simulink model "F16version1"  (R2023b)
settings: Solver=VariableStepAuto  StartTime=0.0  StopTime=60  FixedStep=0.1  RelTol=1e-3
libraries: simulink_extras x4, simulink x2, aerolibasang x2, shared6dof x1, aerolibanim x1
(part 1 of 2)
settings Model: Creator=TADTAWAN  LastModifiedBy=TADTAWAN

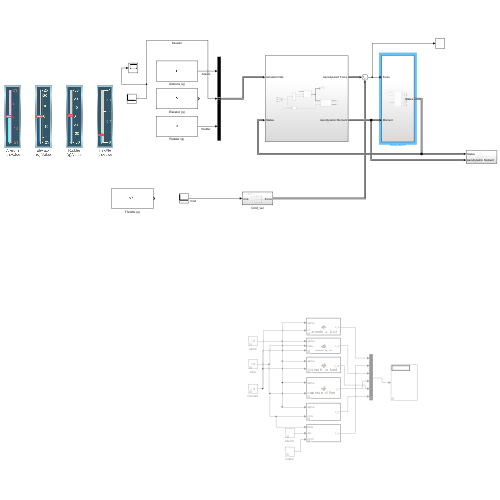
[thumbnail: Simulink's stored preview of the top-level diagram]
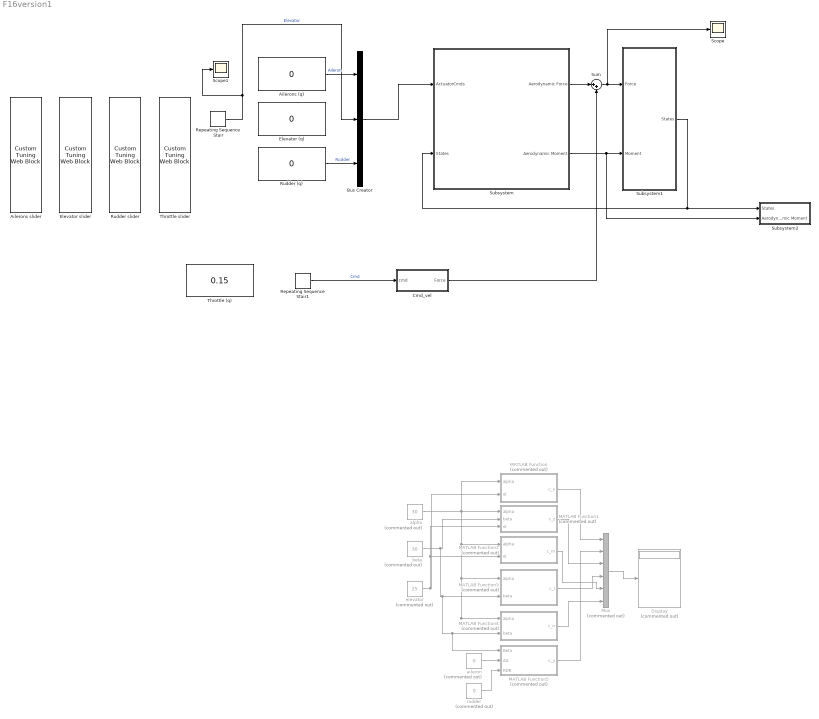
== system F16version1 ==
  Ailerons (q) : Constant  Value=0
  Ailerons slider : CustomTuningWebBlock  LabelPosition=Bottom  ShowInitialText=on  Configuration="{\"components\":[{\"name\":\"LinearScaleComponent\",\"settings\":{\"bounds\":{\"max\":21.5,\"min\":-21.5,\"tickInterval\":\"auto\"},\"internalTickHeightScaleFactor\":0.5,\"labelColor\":[181,82,43],\"labelFont\":{\"font\":\"Arial\",\"fontSize\":12},\"labelOffset\":0.05,\"labelTransparency\":1,\"needleImage\":{\"size\":[596,842],\"src\":\"data:image\\/svg+xml;base64,PD94bWwgdmVyc2lvbj0iMS4wIiBlbmNvZGluZz0idXRmLTgiPz4NCjwhLS0gR2VuZXJhdG9yOiBBZG9iZSBJbGx1c3RyYXRvciAyNS4wLjAsIFNWRyBFeHBvcnQgUGx1Zy1JbiAuIFNWRyBWZXJzaW9uOiA2LjAwIEJ1aWxkIDApICAtLT4NCjxzdmcgdmVyc2lvbj0iMS4xIg0KCSBpZD0ic3ZnOCIgeG1sbnM6Y2M9Imh0dHA6Ly9jcmVhdGl2ZWNvbW1vbnMub3JnL25zIyIgeG1sbnM6ZGM9Imh0dHA6Ly9wdXJsLm9yZy9kYy9lbGVtZW50cy8xLjEvIiB4bWxuczppbmtzY2FwZT0iaHR0cDovL3d3dy5pbmtzY2FwZS5vcmcvbmFtZXNw ...(+2420 chars)\",\"srcOrientation\":\"horizontal\"},\"needleOffset\":[0.0642123287671233,-0.8044596912521441],\"needleSize\":{\"height\":0.07668067226890757,\"width\":0.4337797619047619},\"position\":[0.03623949579831933,0.2829861111111111,0.6088789682539683,0.9196428571428571],\"referencePoint\":\"auto\",\"scaleColors\":[],\"scaleColorsSize\":0.2,\"scaleDirection\":\"BT\",\"showLabels\":1,\"showMinorTicks\":0,\"showSpanLine\":1,\"showTicks\":1,\"tickColor\":[150,61,168],\"tickTransparency\":1,\"valueBarColor\":[15,255,255],\"valueBarOffset\":-0.27,\"valueBarSize\":0.1,\"valueBarTransparency\":1}},{\"name\":\"BackgroundImageComponent\",\"settings\":{\"image\":{\"size\":[380,101],\"src\":\"data:image\\/svg+xml;base64,PHN2ZyB4bWxucz0iaHR0cDovL3d3dy53My5vcmcvMjAwMC9zdmciIHhtbG5zOnhsaW5rPSJodHRwOi8vd3d3LnczLm9yZy8xOTk5L3hsaW5rIiB2aWV3Qm94PSIwIDAgMzgwIDEwMSI+PGRlZnM+PHN0eWxlPi5jbHMtMXtmaWxsOiMwMDJiNDI7fS5jbHMtMntmaWxsOiM0MjcwODI7fS5jbHMtM3tmaWxsOnVybCgjcmFkaWFsLWdyYWRpZW50KTt9LmNscy00e2ZpbGw6I2M4YzhjODtzdHJva2U6IzAwMDt9PC9zdHlsZT48cmFkaWFsR3JhZGllbnQgaWQ9InJhZGlhbC1ncmFkaWVudCIgY3g9IjE5MCIgY3k9IjUwLjUiIHI9IjI2OS4yMSIgZ3JhZGllbnRVbml0cz0idXNlclNwYWNlT25Vc2UiPjxzdG9wIG9mZnNldD0iMC4wMSIgc3RvcC1jb2xvcj0iIzNlNGY1OCIvPjxzdG9wIG9mZnNldD0iMC4wNiIgc3RvcC1jb2xvcj0iIzQ0NTc2MSIvPjxzdG9wIG9mZnNldD0iMC4xNSIgc3RvcC1jb2xvcj0iIzU1NmE3NiIvPjxzdG9wIG9mZnNldD0iMC4yNSIgc3RvcC1jb2xvcj0iIzZkODg5NSIvPjxzdG9wIG9mZnNldD0iMC4zOCIgc3RvcC1jb2xvcj0iIzhmYjJjMyIvPjxzdG9wIG9mZnNldD0iMC41MiIgc3RvcC1jb2xvcj0iI2I2ZTRmYSIvPjxzdG9wIG9mZnNldD0iMSIgc3RvcC1jb2xvcj0iIzE1NDY1NyIvPjwvcmFkaWFsR3JhZGllbnQ+PC9kZWZzPjxnIGlkPSJmcmFtZSI+PGcgaWQ9IkxheWVyXzIiIGRhdGEtbmFtZT0iTGF5ZXIgMiI+PGcgaWQ9IkxheWVyXzEtMiIgZGF0YS1uYW1lPSJMYXllciAxLTIiPjxyZWN0IGlkPSJyZWN0MTAzNiIgY2xhc3M9ImNscy0xIiB4PSIxMSIgeT0iMTEiIHdpZHRoPSIzNTgiIGhlaWdodD0iNzkiLz48cGF0aCBpZD0icGF0aDEwMzgiIGNsYXNzPSJjbHMtMiIgZD0iTTgsOFY5M0gzNzJWOFpNMzY5LDkwSDExVjExSDM2OVoiLz48cGF0aCBpZD0icGF0aDEwNDAiIGNsYXNzPSJjbHMtMyIgZD0iTTAsMFYxMDFIMzgwVjBaTTM3Miw5M0g4VjhIMzcyWiIvPjwvZz48L2c+PC9nPjxnIGlkPSJ0cmFjayI+PHBhdGggaWQ9InJlY3QxNjExIiBjbGFzcz0iY2xzLTQiIGQ9Ik0zMy4zNywyNi41OUgzNDYuNjNjNCwwLDcuMjUsMi42LDcuMjUsNS44MWgwYzAsMy4yMS0zLjI1LDUuODItNy4yNSw1LjgySDMzLjM3Yy00LDAtNy4yNS0yLjYxLTcuMjUtNS44MmgwQzI2LjEyLDI5LjE5LDI5LjM3LDI2LjU5LDMzLjM3LDI2LjU5WiIvPjwvZz48L3N2Zz4=\",\"srcOrientation\":\"horizontal\"},\"position\":[0,0,1,1],\"scaleMode\":\"0\"}},{\"name\":\"ForegroundImageComponent\",\"settings\":{\"image\":{\"size\":[0,0],\"src\":\"default\",\"srcOrientation\":[]},\"isForeground\":1,\"position\":[0,0,1,1],\"scaleMode\":\"0\"}}],\"settings\":{\"BindingType\":\"param\",\"aspectRatio\":3.7777777777777777,\"backgroundColor\":[0,0,0,\"1\"],\"backgroundOffset\":0,\"backgroundOpacity\":1,\"fixedAspectRatio\":\"on\",\"foregroundColor\":[252,252,196],\"orientation\":\"vertical\",\"showBackgroundColor\":false,\"value\":0,\"version\":\"R2023a\"},\"type\":\"LinearGauge\"}"
  Bus Creator : BusCreator  Inputs=3
  Cmd_vel : Subsystem
  Display : Display  Commented=on
  Elevator (q) : Constant  Value=0
  Elevator slider : CustomTuningWebBlock  LabelPosition=Bottom  ShowInitialText=on  Configuration="{\"components\":[{\"name\":\"LinearScaleComponent\",\"settings\":{\"bounds\":{\"max\":25,\"min\":-25,\"tickInterval\":\"auto\"},\"internalTickHeightScaleFactor\":0.5,\"labelColor\":[255,255,200],\"labelFont\":{\"font\":\"Arial\",\"fontSize\":12},\"labelOffset\":0.05,\"labelTransparency\":1,\"needleImage\":{\"size\":[596,842],\"src\":\"data:image\\/svg+xml;base64,PD94bWwgdmVyc2lvbj0iMS4wIiBlbmNvZGluZz0idXRmLTgiPz4NCjwhLS0gR2VuZXJhdG9yOiBBZG9iZSBJbGx1c3RyYXRvciAyNS4wLjAsIFNWRyBFeHBvcnQgUGx1Zy1JbiAuIFNWRyBWZXJzaW9uOiA2LjAwIEJ1aWxkIDApICAtLT4NCjxzdmcgdmVyc2lvbj0iMS4xIg0KCSBpZD0ic3ZnOCIgeG1sbnM6Y2M9Imh0dHA6Ly9jcmVhdGl2ZWNvbW1vbnMub3JnL25zIyIgeG1sbnM6ZGM9Imh0dHA6Ly9wdXJsLm9yZy9kYy9lbGVtZW50cy8xLjEvIiB4bWxuczppbmtzY2FwZT0iaHR0cDovL3d3dy5pbmtzY2FwZS5vcmcvbmFtZXNw ...(+2420 chars)\",\"srcOrientation\":\"horizontal\"},\"needleOffset\":[0.0642123287671233,-0.8044596912521441],\"needleSize\":{\"height\":0.07668067226890757,\"width\":0.4337797619047619},\"position\":[0.03623949579831933,0.2829861111111111,0.6088789682539683,0.9196428571428571],\"referencePoint\":\"auto\",\"scaleColors\":[],\"scaleColorsSize\":0.2,\"scaleDirection\":\"BT\",\"showLabels\":1,\"showMinorTicks\":0,\"showSpanLine\":1,\"showTicks\":1,\"tickColor\":[252,252,197],\"tickTransparency\":1,\"valueBarColor\":[0,114,189],\"valueBarOffset\":-0.27,\"valueBarSize\":0.1,\"valueBarTransparency\":1}},{\"name\":\"BackgroundImageComponent\",\"settings\":{\"image\":{\"size\":[380,101],\"src\":\"data:image\\/svg+xml;base64,PHN2ZyB4bWxucz0iaHR0cDovL3d3dy53My5vcmcvMjAwMC9zdmciIHhtbG5zOnhsaW5rPSJodHRwOi8vd3d3LnczLm9yZy8xOTk5L3hsaW5rIiB2aWV3Qm94PSIwIDAgMzgwIDEwMSI+PGRlZnM+PHN0eWxlPi5jbHMtMXtmaWxsOiMwMDJiNDI7fS5jbHMtMntmaWxsOiM0MjcwODI7fS5jbHMtM3tmaWxsOnVybCgjcmFkaWFsLWdyYWRpZW50KTt9LmNscy00e2ZpbGw6I2M4YzhjODtzdHJva2U6IzAwMDt9PC9zdHlsZT48cmFkaWFsR3JhZGllbnQgaWQ9InJhZGlhbC1ncmFkaWVudCIgY3g9IjE5MCIgY3k9IjUwLjUiIHI9IjI2OS4yMSIgZ3JhZGllbnRVbml0cz0idXNlclNwYWNlT25Vc2UiPjxzdG9wIG9mZnNldD0iMC4wMSIgc3RvcC1jb2xvcj0iIzNlNGY1OCIvPjxzdG9wIG9mZnNldD0iMC4wNiIgc3RvcC1jb2xvcj0iIzQ0NTc2MSIvPjxzdG9wIG9mZnNldD0iMC4xNSIgc3RvcC1jb2xvcj0iIzU1NmE3NiIvPjxzdG9wIG9mZnNldD0iMC4yNSIgc3RvcC1jb2xvcj0iIzZkODg5NSIvPjxzdG9wIG9mZnNldD0iMC4zOCIgc3RvcC1jb2xvcj0iIzhmYjJjMyIvPjxzdG9wIG9mZnNldD0iMC41MiIgc3RvcC1jb2xvcj0iI2I2ZTRmYSIvPjxzdG9wIG9mZnNldD0iMSIgc3RvcC1jb2xvcj0iIzE1NDY1NyIvPjwvcmFkaWFsR3JhZGllbnQ+PC9kZWZzPjxnIGlkPSJmcmFtZSI+PGcgaWQ9IkxheWVyXzIiIGRhdGEtbmFtZT0iTGF5ZXIgMiI+PGcgaWQ9IkxheWVyXzEtMiIgZGF0YS1uYW1lPSJMYXllciAxLTIiPjxyZWN0IGlkPSJyZWN0MTAzNiIgY2xhc3M9ImNscy0xIiB4PSIxMSIgeT0iMTEiIHdpZHRoPSIzNTgiIGhlaWdodD0iNzkiLz48cGF0aCBpZD0icGF0aDEwMzgiIGNsYXNzPSJjbHMtMiIgZD0iTTgsOFY5M0gzNzJWOFpNMzY5LDkwSDExVjExSDM2OVoiLz48cGF0aCBpZD0icGF0aDEwNDAiIGNsYXNzPSJjbHMtMyIgZD0iTTAsMFYxMDFIMzgwVjBaTTM3Miw5M0g4VjhIMzcyWiIvPjwvZz48L2c+PC9nPjxnIGlkPSJ0cmFjayI+PHBhdGggaWQ9InJlY3QxNjExIiBjbGFzcz0iY2xzLTQiIGQ9Ik0zMy4zNywyNi41OUgzNDYuNjNjNCwwLDcuMjUsMi42LDcuMjUsNS44MWgwYzAsMy4yMS0zLjI1LDUuODItNy4yNSw1LjgySDMzLjM3Yy00LDAtNy4yNS0yLjYxLTcuMjUtNS44MmgwQzI2LjEyLDI5LjE5LDI5LjM3LDI2LjU5LDMzLjM3LDI2LjU5WiIvPjwvZz48L3N2Zz4=\",\"srcOrientation\":\"horizontal\"},\"position\":[0,0,1,1],\"scaleMode\":\"0\"}},{\"name\":\"ForegroundImageComponent\",\"settings\":{\"image\":{\"size\":[0,0],\"src\":\"default\",\"srcOrientation\":[]},\"isForeground\":1,\"position\":[0,0,1,1],\"scaleMode\":\"0\"}}],\"settings\":{\"BindingType\":\"param\",\"aspectRatio\":3.7777777777777777,\"backgroundColor\":[0,0,0,\"1\"],\"backgroundOffset\":0,\"backgroundOpacity\":1,\"fixedAspectRatio\":\"on\",\"foregroundColor\":[252,252,196],\"orientation\":\"vertical\",\"showBackgroundColor\":false,\"value\":0,\"version\":\"R2023a\"},\"type\":\"LinearGauge\"}"
  MATLAB Function : MATLAB Function  Commented=on  TreatAsAtomicUnit=on
  MATLAB Function1 : MATLAB Function  Commented=on  TreatAsAtomicUnit=on
  MATLAB Function2 : MATLAB Function  Commented=on  TreatAsAtomicUnit=on
  MATLAB Function3 : MATLAB Function  Commented=on  TreatAsAtomicUnit=on
  MATLAB Function4 : MATLAB Function  Commented=on  TreatAsAtomicUnit=on
  MATLAB Function5 : MATLAB Function  Commented=on  TreatAsAtomicUnit=on
  Mux : Mux  Commented=on  Inputs=6
  Repeating Sequence Stair : simulink/Sources/Repeating Sequence Stair  OutValues=[-1.5].'  tsamp=10  OutMin=[]  OutMax=[]  OutDataTypeStr=double  OutputDataTypeScalingMode=double  OutDataType=fixdt(0,8)  ConRadixGroup=Best Precision: Vector-wise  OutScaling=2^-12
  Repeating Sequence Stair1 : simulink/Sources/Repeating Sequence Stair  OutValues=[0.5].'  tsamp=10  OutMin=[]  OutMax=[]  OutDataTypeStr=double  OutputDataTypeScalingMode=double  OutDataType=fixdt(0,8)  ConRadixGroup=Best Precision: Vector-wise  OutScaling=2^-12
  Rudder (q) : Constant  Value=0
  Rudder slider : CustomTuningWebBlock  LabelPosition=Bottom  ShowInitialText=on  Configuration="{\"components\":[{\"name\":\"LinearScaleComponent\",\"settings\":{\"bounds\":{\"max\":30,\"min\":-30,\"tickInterval\":\"auto\"},\"internalTickHeightScaleFactor\":0.5,\"labelColor\":[255,255,200],\"labelFont\":{\"font\":\"Arial\",\"fontSize\":12},\"labelOffset\":0.05,\"labelTransparency\":1,\"needleImage\":{\"size\":[596,842],\"src\":\"data:image\\/svg+xml;base64,PD94bWwgdmVyc2lvbj0iMS4wIiBlbmNvZGluZz0idXRmLTgiPz4NCjwhLS0gR2VuZXJhdG9yOiBBZG9iZSBJbGx1c3RyYXRvciAyNS4wLjAsIFNWRyBFeHBvcnQgUGx1Zy1JbiAuIFNWRyBWZXJzaW9uOiA2LjAwIEJ1aWxkIDApICAtLT4NCjxzdmcgdmVyc2lvbj0iMS4xIg0KCSBpZD0ic3ZnOCIgeG1sbnM6Y2M9Imh0dHA6Ly9jcmVhdGl2ZWNvbW1vbnMub3JnL25zIyIgeG1sbnM6ZGM9Imh0dHA6Ly9wdXJsLm9yZy9kYy9lbGVtZW50cy8xLjEvIiB4bWxuczppbmtzY2FwZT0iaHR0cDovL3d3dy5pbmtzY2FwZS5vcmcvbmFtZXNw ...(+2420 chars)\",\"srcOrientation\":\"Right\"},\"needleOffset\":[-0.21513706793802145,-0.7877922077922078],\"needleSize\":{\"height\":0.07666301169590643,\"width\":0.43370508054522927},\"position\":[0.03623949579831933,0.2829861111111111,0.6088789682539683,0.9196428571428571],\"referencePoint\":\"auto\",\"scaleColors\":[],\"scaleColorsSize\":0.2,\"scaleDirection\":\"BT\",\"showLabels\":1,\"showMinorTicks\":0,\"showSpanLine\":1,\"showTicks\":1,\"tickColor\":[252,252,197],\"tickTransparency\":1,\"valueBarColor\":[0,114,189],\"valueBarOffset\":-0.27,\"valueBarSize\":0.1,\"valueBarTransparency\":1}},{\"name\":\"BackgroundImageComponent\",\"settings\":{\"image\":{\"size\":[380,101],\"src\":\"data:image\\/svg+xml;base64,PHN2ZyB4bWxucz0iaHR0cDovL3d3dy53My5vcmcvMjAwMC9zdmciIHhtbG5zOnhsaW5rPSJodHRwOi8vd3d3LnczLm9yZy8xOTk5L3hsaW5rIiB2aWV3Qm94PSIwIDAgMzgwIDEwMSI+PGRlZnM+PHN0eWxlPi5jbHMtMXtmaWxsOiMwMDJiNDI7fS5jbHMtMntmaWxsOiM0MjcwODI7fS5jbHMtM3tmaWxsOnVybCgjcmFkaWFsLWdyYWRpZW50KTt9LmNscy00e2ZpbGw6I2M4YzhjODtzdHJva2U6IzAwMDt9PC9zdHlsZT48cmFkaWFsR3JhZGllbnQgaWQ9InJhZGlhbC1ncmFkaWVudCIgY3g9IjE5MCIgY3k9IjUwLjUiIHI9IjI2OS4yMSIgZ3JhZGllbnRVbml0cz0idXNlclNwYWNlT25Vc2UiPjxzdG9wIG9mZnNldD0iMC4wMSIgc3RvcC1jb2xvcj0iIzNlNGY1OCIvPjxzdG9wIG9mZnNldD0iMC4wNiIgc3RvcC1jb2xvcj0iIzQ0NTc2MSIvPjxzdG9wIG9mZnNldD0iMC4xNSIgc3RvcC1jb2xvcj0iIzU1NmE3NiIvPjxzdG9wIG9mZnNldD0iMC4yNSIgc3RvcC1jb2xvcj0iIzZkODg5NSIvPjxzdG9wIG9mZnNldD0iMC4zOCIgc3RvcC1jb2xvcj0iIzhmYjJjMyIvPjxzdG9wIG9mZnNldD0iMC41MiIgc3RvcC1jb2xvcj0iI2I2ZTRmYSIvPjxzdG9wIG9mZnNldD0iMSIgc3RvcC1jb2xvcj0iIzE1NDY1NyIvPjwvcmFkaWFsR3JhZGllbnQ+PC9kZWZzPjxnIGlkPSJmcmFtZSI+PGcgaWQ9IkxheWVyXzIiIGRhdGEtbmFtZT0iTGF5ZXIgMiI+PGcgaWQ9IkxheWVyXzEtMiIgZGF0YS1uYW1lPSJMYXllciAxLTIiPjxyZWN0IGlkPSJyZWN0MTAzNiIgY2xhc3M9ImNscy0xIiB4PSIxMSIgeT0iMTEiIHdpZHRoPSIzNTgiIGhlaWdodD0iNzkiLz48cGF0aCBpZD0icGF0aDEwMzgiIGNsYXNzPSJjbHMtMiIgZD0iTTgsOFY5M0gzNzJWOFpNMzY5LDkwSDExVjExSDM2OVoiLz48cGF0aCBpZD0icGF0aDEwNDAiIGNsYXNzPSJjbHMtMyIgZD0iTTAsMFYxMDFIMzgwVjBaTTM3Miw5M0g4VjhIMzcyWiIvPjwvZz48L2c+PC9nPjxnIGlkPSJ0cmFjayI+PHBhdGggaWQ9InJlY3QxNjExIiBjbGFzcz0iY2xzLTQiIGQ9Ik0zMy4zNywyNi41OUgzNDYuNjNjNCwwLDcuMjUsMi42LDcuMjUsNS44MWgwYzAsMy4yMS0zLjI1LDUuODItNy4yNSw1LjgySDMzLjM3Yy00LDAtNy4yNS0yLjYxLTcuMjUtNS44MmgwQzI2LjEyLDI5LjE5LDI5LjM3LDI2LjU5LDMzLjM3LDI2LjU5WiIvPjwvZz48L3N2Zz4=\",\"srcOrientation\":\"horizontal\"},\"position\":[0,0,1,1],\"scaleMode\":\"0\"}},{\"name\":\"ForegroundImageComponent\",\"settings\":{\"image\":{\"size\":[0,0],\"src\":\"default\",\"srcOrientation\":[]},\"isForeground\":1,\"position\":[0,0,1,1],\"scaleMode\":\"0\"}}],\"settings\":{\"BindingType\":\"param\",\"aspectRatio\":3.7777777777777777,\"backgroundColor\":[0,0,0,\"1\"],\"backgroundOffset\":0,\"backgroundOpacity\":1,\"fixedAspectRatio\":\"on\",\"foregroundColor\":[252,252,196],\"orientation\":\"vertical\",\"showBackgroundColor\":false,\"value\":0,\"version\":\"R2023a\"},\"type\":\"LinearGauge\"}"
  Scope : Scope
  Scope1 : Scope
  Subsystem : Subsystem
  Subsystem1 : Subsystem
  Subsystem2 : Subsystem
  Sum : Sum  Inputs=|++
  Throttle (q) : Constant  Value=0.15
  Throttle slider : CustomTuningWebBlock  LabelPosition=Bottom  ShowInitialText=on  Configuration="{\"components\":[{\"name\":\"LinearScaleComponent\",\"settings\":{\"bounds\":{\"max\":1,\"min\":0,\"tickInterval\":\"auto\"},\"internalTickHeightScaleFactor\":0.5,\"labelColor\":[255,255,200],\"labelFont\":{\"font\":\"Arial\",\"fontSize\":12},\"labelOffset\":0.05,\"labelTransparency\":1,\"needleImage\":{\"size\":[596,842],\"src\":\"data:image\\/svg+xml;base64,PD94bWwgdmVyc2lvbj0iMS4wIiBlbmNvZGluZz0idXRmLTgiPz4NCjwhLS0gR2VuZXJhdG9yOiBBZG9iZSBJbGx1c3RyYXRvciAyNS4wLjAsIFNWRyBFeHBvcnQgUGx1Zy1JbiAuIFNWRyBWZXJzaW9uOiA2LjAwIEJ1aWxkIDApICAtLT4NCjxzdmcgdmVyc2lvbj0iMS4xIg0KCSBpZD0ic3ZnOCIgeG1sbnM6Y2M9Imh0dHA6Ly9jcmVhdGl2ZWNvbW1vbnMub3JnL25zIyIgeG1sbnM6ZGM9Imh0dHA6Ly9wdXJsLm9yZy9kYy9lbGVtZW50cy8xLjEvIiB4bWxuczppbmtzY2FwZT0iaHR0cDovL3d3dy5pbmtzY2FwZS5vcmcvbmFtZXNw ...(+2420 chars)\",\"srcOrientation\":\"horizontal\"},\"needleOffset\":[0.0642123287671233,-0.8044596912521441],\"needleSize\":{\"height\":0.07668067226890757,\"width\":0.4337797619047619},\"position\":[0.03623949579831933,0.2829861111111111,0.6088789682539683,0.9196428571428571],\"referencePoint\":\"auto\",\"scaleColors\":[],\"scaleColorsSize\":0.2,\"scaleDirection\":\"BT\",\"showLabels\":1,\"showMinorTicks\":0,\"showSpanLine\":1,\"showTicks\":1,\"tickColor\":[252,252,197],\"tickTransparency\":1,\"valueBarColor\":[0,114,189],\"valueBarOffset\":-0.27,\"valueBarSize\":0.1,\"valueBarTransparency\":1}},{\"name\":\"BackgroundImageComponent\",\"settings\":{\"image\":{\"size\":[380,101],\"src\":\"data:image\\/svg+xml;base64,PHN2ZyB4bWxucz0iaHR0cDovL3d3dy53My5vcmcvMjAwMC9zdmciIHhtbG5zOnhsaW5rPSJodHRwOi8vd3d3LnczLm9yZy8xOTk5L3hsaW5rIiB2aWV3Qm94PSIwIDAgMzgwIDEwMSI+PGRlZnM+PHN0eWxlPi5jbHMtMXtmaWxsOiMwMDJiNDI7fS5jbHMtMntmaWxsOiM0MjcwODI7fS5jbHMtM3tmaWxsOnVybCgjcmFkaWFsLWdyYWRpZW50KTt9LmNscy00e2ZpbGw6I2M4YzhjODtzdHJva2U6IzAwMDt9PC9zdHlsZT48cmFkaWFsR3JhZGllbnQgaWQ9InJhZGlhbC1ncmFkaWVudCIgY3g9IjE5MCIgY3k9IjUwLjUiIHI9IjI2OS4yMSIgZ3JhZGllbnRVbml0cz0idXNlclNwYWNlT25Vc2UiPjxzdG9wIG9mZnNldD0iMC4wMSIgc3RvcC1jb2xvcj0iIzNlNGY1OCIvPjxzdG9wIG9mZnNldD0iMC4wNiIgc3RvcC1jb2xvcj0iIzQ0NTc2MSIvPjxzdG9wIG9mZnNldD0iMC4xNSIgc3RvcC1jb2xvcj0iIzU1NmE3NiIvPjxzdG9wIG9mZnNldD0iMC4yNSIgc3RvcC1jb2xvcj0iIzZkODg5NSIvPjxzdG9wIG9mZnNldD0iMC4zOCIgc3RvcC1jb2xvcj0iIzhmYjJjMyIvPjxzdG9wIG9mZnNldD0iMC41MiIgc3RvcC1jb2xvcj0iI2I2ZTRmYSIvPjxzdG9wIG9mZnNldD0iMSIgc3RvcC1jb2xvcj0iIzE1NDY1NyIvPjwvcmFkaWFsR3JhZGllbnQ+PC9kZWZzPjxnIGlkPSJmcmFtZSI+PGcgaWQ9IkxheWVyXzIiIGRhdGEtbmFtZT0iTGF5ZXIgMiI+PGcgaWQ9IkxheWVyXzEtMiIgZGF0YS1uYW1lPSJMYXllciAxLTIiPjxyZWN0IGlkPSJyZWN0MTAzNiIgY2xhc3M9ImNscy0xIiB4PSIxMSIgeT0iMTEiIHdpZHRoPSIzNTgiIGhlaWdodD0iNzkiLz48cGF0aCBpZD0icGF0aDEwMzgiIGNsYXNzPSJjbHMtMiIgZD0iTTgsOFY5M0gzNzJWOFpNMzY5LDkwSDExVjExSDM2OVoiLz48cGF0aCBpZD0icGF0aDEwNDAiIGNsYXNzPSJjbHMtMyIgZD0iTTAsMFYxMDFIMzgwVjBaTTM3Miw5M0g4VjhIMzcyWiIvPjwvZz48L2c+PC9nPjxnIGlkPSJ0cmFjayI+PHBhdGggaWQ9InJlY3QxNjExIiBjbGFzcz0iY2xzLTQiIGQ9Ik0zMy4zNywyNi41OUgzNDYuNjNjNCwwLDcuMjUsMi42LDcuMjUsNS44MWgwYzAsMy4yMS0zLjI1LDUuODItNy4yNSw1LjgySDMzLjM3Yy00LDAtNy4yNS0yLjYxLTcuMjUtNS44MmgwQzI2LjEyLDI5LjE5LDI5LjM3LDI2LjU5LDMzLjM3LDI2LjU5WiIvPjwvZz48L3N2Zz4=\",\"srcOrientation\":\"horizontal\"},\"position\":[0,0,1,1],\"scaleMode\":\"0\"}},{\"name\":\"ForegroundImageComponent\",\"settings\":{\"image\":{\"size\":[0,0],\"src\":\"default\",\"srcOrientation\":[]},\"isForeground\":1,\"position\":[0,0,1,1],\"scaleMode\":\"0\"}}],\"settings\":{\"BindingType\":\"param\",\"aspectRatio\":3.7777777777777777,\"backgroundColor\":[0,0,0,\"1\"],\"backgroundOffset\":0,\"backgroundOpacity\":1,\"fixedAspectRatio\":\"on\",\"foregroundColor\":[252,252,196],\"orientation\":\"vertical\",\"showBackgroundColor\":false,\"value\":0,\"version\":\"R2023a\"},\"type\":\"LinearGauge\"}"
  aileron : Constant  Commented=on  Value=0
  alpha : Constant  Commented=on  Value=30
  beta : Constant  Commented=on  Value=30
  elevator : Constant  Commented=on  Value=25
  rudder : Constant  Commented=on  Value=0
  wires:
  Ailerons (q)/1 -> Bus Creator/1  "Aileron"
  Rudder (q)/1 -> Bus Creator/3  "Rudder"
  Bus Creator/1 -> Subsystem/1(ActuatorCmds)
  Subsystem/1(Aerodynamic Force) -> Sum/1
  Subsystem/2(Aerodynamic Moment) -> Subsystem2/2(Aerodynamic Moment), Subsystem1/2(Moment)
  Cmd_vel/1(Force) -> Sum/2
  Sum/1 -> Scope/1, Subsystem1/1(Force)
  Subsystem1/1(States) -> Subsystem/2(States), Subsystem2/1(States)
  alpha/1 -> MATLAB Function4/1(alpha), MATLAB Function3/1(alpha), MATLAB Function2/1(alpha), MATLAB Function1/1(alpha), MATLAB Function/1(alpha)
  beta/1 -> MATLAB Function5/1(Beta), MATLAB Function4/2(beta), MATLAB Function3/2(beta), MATLAB Function1/2(beta)
  elevator/1 -> MATLAB Function2/2(el), MATLAB Function1/3(el), MATLAB Function/2(el)
  aileron/1 -> MATLAB Function5/2(AIL)
  rudder/1 -> MATLAB Function5/3(RDR)
  MATLAB Function/1(c_x) -> Mux/1
  MATLAB Function5/1(c_y) -> Mux/2
  MATLAB Function1/1(c_z) -> Mux/3
  MATLAB Function3/1(c_l) -> Mux/4
  MATLAB Function2/1(c_m) -> Mux/5
  MATLAB Function4/1(c_n) -> Mux/6
  Mux/1 -> Display/1
  Repeating Sequence Stair/1 -> Scope1/1, Bus Creator/2  "Elevator"
  Repeating Sequence Stair1/1 -> Cmd_vel/1(cmd)  "Cmd"

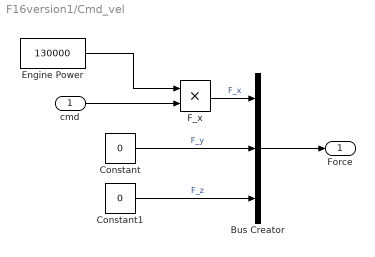
== system F16version1/Cmd_vel ==
  cmd : Inport
  Bus Creator : BusCreator  Inputs=3
  Constant : Constant  Value=0
  Constant1 : Constant  Value=0
  Engine Power : Constant  Value=130000
  F_x : Product
  Force : Outport
  wires:
  Engine Power/1 -> F_x/1
  cmd/1 -> F_x/2
  F_x/1 -> Bus Creator/1  "F_x"
  Constant/1 -> Bus Creator/2  "F_y"
  Constant1/1 -> Bus Creator/3  "F_z"
  Bus Creator/1 -> Force/1

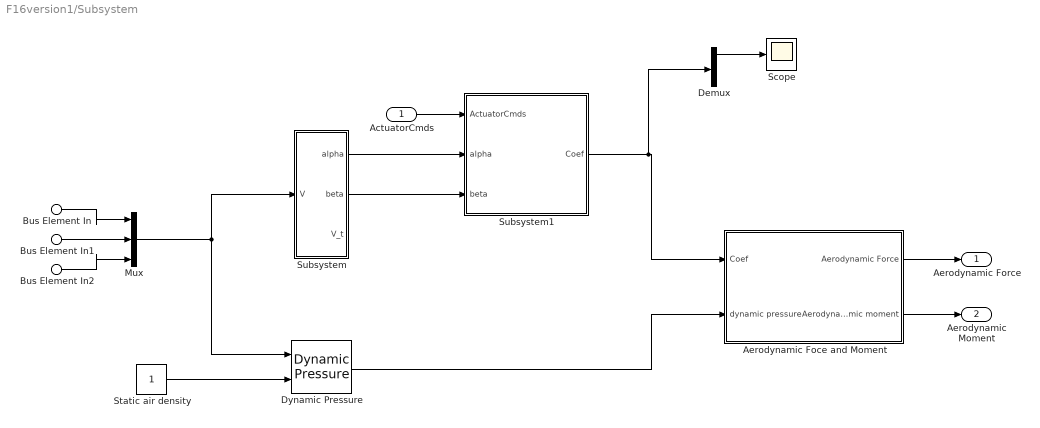
== system F16version1/Subsystem ==
  ActuatorCmds : Inport
  Bus Element In : Inport  Port=2  PortName=States  Element=U
  Bus Element In1 : Inport  Port=2  PortName=States  Element=V
  Bus Element In2 : Inport  Port=2  PortName=States  Element=W
  Aerodynamic Foce and Moment : Subsystem
  Demux : Demux  Outputs=6
  Dynamic Pressure : aerolibasang/Dynamic Pressure
  Mux : Mux  Inputs=3
  Scope : Scope
  Static air density : Constant
  Subsystem : Subsystem
  Subsystem1 : Subsystem
  Aerodynamic Force : Outport
  Aerodynamic Moment : Outport  Port=2
  wires:
  Bus Element In1/1 -> Mux/2
  Bus Element In/1 -> Mux/1
  Bus Element In2/1 -> Mux/3
  Mux/1 -> Dynamic Pressure/1, Subsystem/1(V)
  ActuatorCmds/1 -> Subsystem1/1(ActuatorCmds)
  Subsystem/1(alpha) -> Subsystem1/2(alpha)
  Subsystem/2(beta) -> Subsystem1/3(beta)
  Static air density/1 -> Dynamic Pressure/2
  Dynamic Pressure/1 -> Aerodynamic Foce and Moment/2(dynamic pressure)
  Subsystem1/1(Coef) -> Demux/1, Aerodynamic Foce and Moment/1(Coef)
  Aerodynamic Foce and Moment/1(Aerodynamic Force) -> Aerodynamic Force/1
  Aerodynamic Foce and Moment/2(Aerodynamic moment) -> Aerodynamic Moment/1
  Demux/1 -> Scope/1

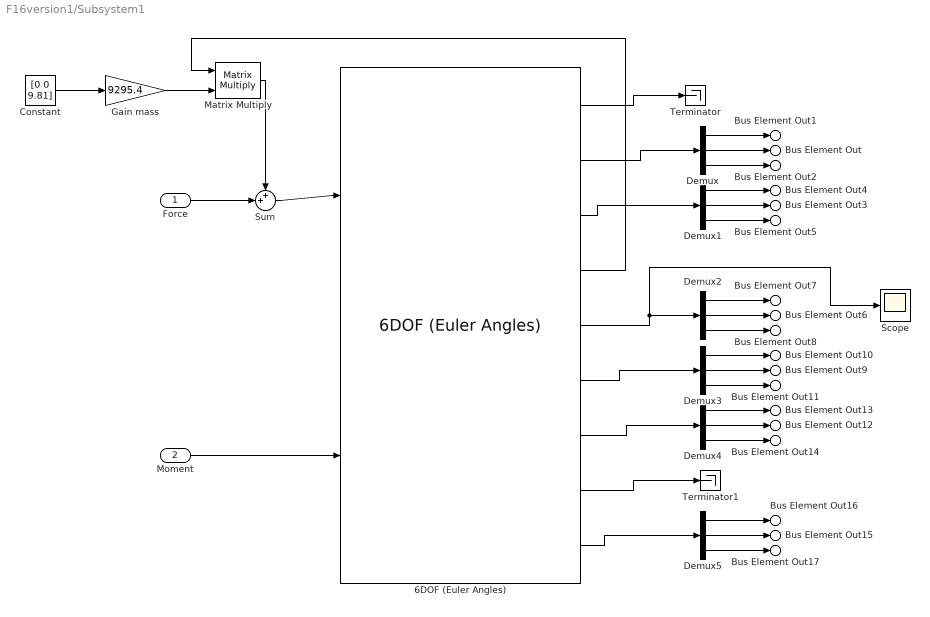
== system F16version1/Subsystem1 ==
  Force : Inport
  Moment : Inport  Port=2
  6DOF (Euler Angles) : shared6dof/6DOF (Euler Angles)  units=Metric (MKS)  mtype=Fixed  rep=Euler Angles  xme_0=[0, 0,-2000]  Vm_0=[0.01, 0.01, 0.01]  eul_0=[0.0, 0.0, 0]  pm_0=[0, 0, 0]  mass_0=91188/9.81  mass_e=0.5  mass_f=2.0  inertia=|  inertia_e=eye(3)  inertia_f=2*eye(3)  k_quat=1.0  vre_flag=off  abi_flag=on  aMode=0  xme_statename={'Xe', 'Ye', 'Ze'}  Vm_statename={'U', 'V', 'W'}  eul_statename={'phi', 'theta', 'psi'}  quat_statename=''  pm_statename={'p', 'q', 'r'}  mass_statename=''
      | [12881.4, 0, 1522.0;
      |  0, 75696.9, 0;
      |  1522.0, 0, 85557.2]
  Constant : Constant  Value=[0 0 9.81]
  Demux{,1..5} (6 alike) : Demux  Outputs=3
  Gain mass : Gain  Gain=9295.4
  Matrix Multiply : Product  Multiplication=Matrix(*)
  Scope : Scope
  Sum : Sum  Inputs=++|
  Terminator : Terminator
  Terminator1 : Terminator
  Bus Element Out : Outport  PortName=States  Element=Ye
  Bus Element Out1 : Outport  PortName=States  Element=Xe
  Bus Element Out2 : Outport  PortName=States  Element=Ze
  Bus Element Out3 : Outport  PortName=States  Element=theta
  Bus Element Out4 : Outport  PortName=States  Element=phi
  Bus Element Out5 : Outport  PortName=States  Element=psi
  Bus Element Out6 : Outport  PortName=States  Element=V
  Bus Element Out7 : Outport  PortName=States  Element=U
  Bus Element Out8 : Outport  PortName=States  Element=W
  Bus Element Out9 : Outport  PortName=States  Element=q
  Bus Element Out10 : Outport  PortName=States  Element=p
  Bus Element Out11 : Outport  PortName=States  Element=r
  Bus Element Out12 : Outport  PortName=States  Element=q_dot
  Bus Element Out13 : Outport  PortName=States  Element=p_dot
  Bus Element Out14 : Outport  PortName=States  Element=r_dot
  Bus Element Out15 : Outport  PortName=States  Element=Aye
  Bus Element Out16 : Outport  PortName=States  Element=Axe
  Bus Element Out17 : Outport  PortName=States  Element=Aze
  wires:
  Moment/1 -> 6DOF (Euler Angles)/2
  Force/1 -> Sum/2
  Constant/1 -> Gain mass/1
  Gain mass/1 -> Matrix Multiply/2
  Matrix Multiply/1 -> Sum/1
  Sum/1 -> 6DOF (Euler Angles)/1
  6DOF (Euler Angles)/4 -> Matrix Multiply/1
  6DOF (Euler Angles)/2 -> Demux/1
  Demux/2 -> Bus Element Out/1
  Demux/1 -> Bus Element Out1/1
  Demux/3 -> Bus Element Out2/1
  Demux1/3 -> Bus Element Out5/1
  Demux1/2 -> Bus Element Out3/1
  Demux1/1 -> Bus Element Out4/1
  6DOF (Euler Angles)/3 -> Demux1/1
  Demux2/1 -> Bus Element Out7/1
  Demux2/3 -> Bus Element Out8/1
  Demux2/2 -> Bus Element Out6/1
  6DOF (Euler Angles)/5 -> Scope/1, Demux2/1
  Demux3/1 -> Bus Element Out10/1
  Demux3/3 -> Bus Element Out11/1
  Demux3/2 -> Bus Element Out9/1
  6DOF (Euler Angles)/6 -> Demux3/1
  Demux4/1 -> Bus Element Out13/1
  Demux4/3 -> Bus Element Out14/1
  Demux4/2 -> Bus Element Out12/1
  6DOF (Euler Angles)/7 -> Demux4/1
  Demux5/1 -> Bus Element Out16/1
  Demux5/3 -> Bus Element Out17/1
  Demux5/2 -> Bus Element Out15/1
  6DOF (Euler Angles)/1 -> Terminator/1
  6DOF (Euler Angles)/8 -> Terminator1/1
  6DOF (Euler Angles)/9 -> Demux5/1

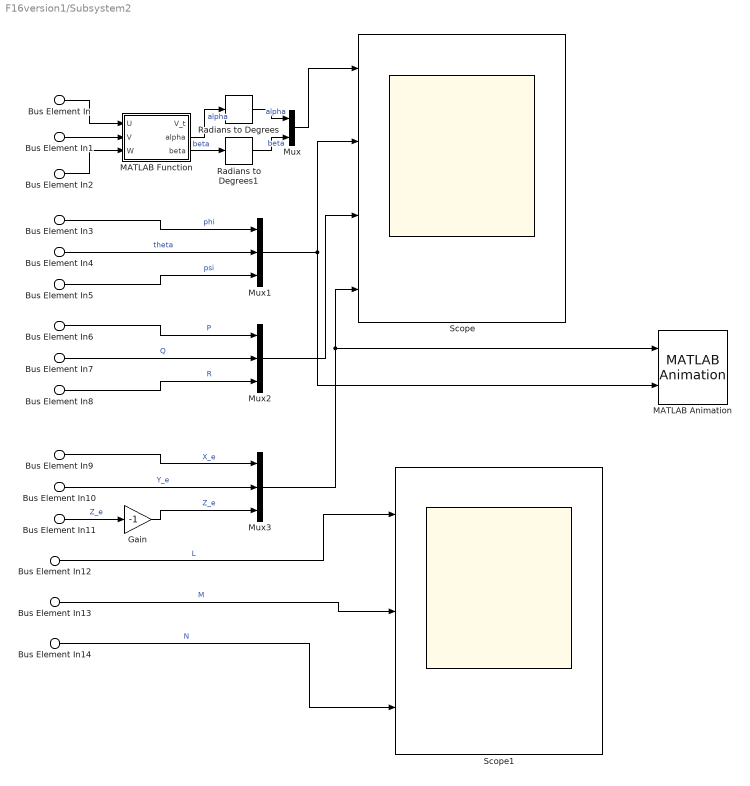
== system F16version1/Subsystem2 ==
  Bus Element In : Inport  PortName=States  Element=U
  Bus Element In2 : Inport  PortName=States  Element=W
  Bus Element In1 : Inport  PortName=States  Element=V
  Bus Element In3 : Inport  PortName=States  Element=phi
  Bus Element In4 : Inport  PortName=States  Element=theta
  Bus Element In5 : Inport  PortName=States  Element=psi
  Bus Element In6 : Inport  PortName=States  Element=p
  Bus Element In7 : Inport  PortName=States  Element=q
  Bus Element In8 : Inport  PortName=States  Element=r
  Bus Element In9 : Inport  PortName=States  Element=Xe
  Bus Element In10 : Inport  PortName=States  Element=Ye
  Bus Element In11 : Inport  PortName=States  Element=Ze
  Bus Element In12 : Inport  Port=2  PortName=Aerodynamic Moment  Element=L
  Bus Element In13 : Inport  Port=2  PortName=Aerodynamic Moment  Element=M
  Bus Element In14 : Inport  Port=2  PortName=Aerodynamic Moment  Element=N
  Gain : Gain  Gain=-1
  MATLAB Animation : aerolibanim/MATLAB Animation  Tag=Matlab Animation 6 DOF  Vehicles=1  Geometries='astredwedge.mat'  BoundingBoxCoordinates=[-50,50,-50,50,-50,50]  CameraOffset=[-150,-50,0]  CameraViewAngle=3  SampleTime=0.2  FigurePosition=[-1020,327,559,396]
  MATLAB Function : MATLAB Function  TreatAsAtomicUnit=on
  Mux : Mux  Inputs=2
  Mux1 : Mux  Inputs=3
  Mux2 : Mux  Inputs=3
  Mux3 : Mux  Inputs=3
  Radians to Degrees : simulink_extras/Transformations/Radians to Degrees
  Radians to Degrees1 : simulink_extras/Transformations/Radians to Degrees
  Scope : Scope  NumInputPorts=4
  Scope1 : Scope  NumInputPorts=3
  wires:
  Bus Element In/1 -> MATLAB Function/1(U)
  Bus Element In1/1 -> MATLAB Function/2(V)
  Bus Element In2/1 -> MATLAB Function/3(W)
  MATLAB Function/2(alpha) -> Radians to Degrees/1  "alpha"
  MATLAB Function/3(beta) -> Radians to Degrees1/1  "beta"
  Mux/1 -> Scope/1
  Bus Element In4/1 -> Mux1/2  "theta"
  Bus Element In3/1 -> Mux1/1  "phi"
  Bus Element In5/1 -> Mux1/3  "psi"
  Mux1/1 -> MATLAB Animation/2, Scope/2
  Bus Element In8/1 -> Mux2/3  "R"
  Bus Element In7/1 -> Mux2/2  "Q"
  Mux2/1 -> Scope/3
  Bus Element In6/1 -> Mux2/1  "P"
  Bus Element In11/1 -> Gain/1  "Z_e"
  Bus Element In10/1 -> Mux3/2  "Y_e"
  Bus Element In9/1 -> Mux3/1  "X_e"
  Mux3/1 -> MATLAB Animation/1, Scope/4
  Bus Element In13/1 -> Scope1/2  "M"
  Bus Element In12/1 -> Scope1/1  "L"
  Bus Element In14/1 -> Scope1/3  "N"
  Radians to Degrees/1 -> Mux/1  "alpha"
  Radians to Degrees1/1 -> Mux/2  "beta"
  Gain/1 -> Mux3/3  "Z_e"

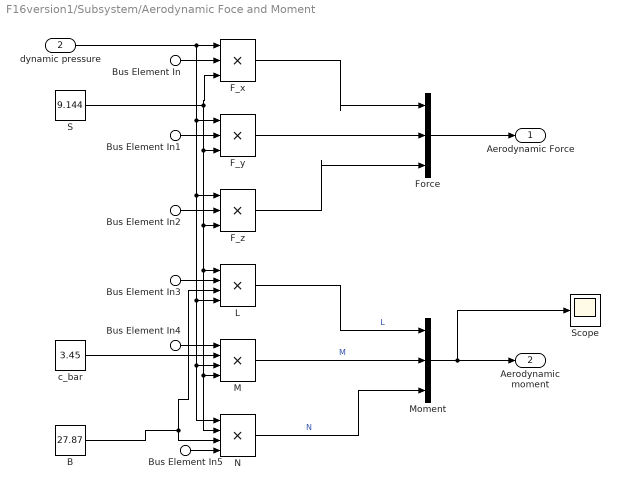
== system F16version1/Subsystem/Aerodynamic Foce and Moment ==
  Bus Element In : Inport  PortName=Coef  Element=c_x
  Bus Element In1 : Inport  PortName=Coef  Element=c_y
  Bus Element In2 : Inport  PortName=Coef  Element=c_z
  Bus Element In3 : Inport  PortName=Coef  Element=c_l
  Bus Element In4 : Inport  PortName=Coef  Element=c_m
  Bus Element In5 : Inport  PortName=Coef  Element=c_n
  dynamic pressure : Inport  Port=2
  B : Constant  Value=27.87
  F_x : Product  Inputs=3
  F_y : Product  Inputs=3
  F_z : Product  Inputs=3
  Force : BusCreator  Inputs=3
  L : Product  Inputs=4
  M : Product  Inputs=4
  Moment : BusCreator  Inputs=3
  N : Product  Inputs=4
  S : Constant  Value=9.144
  Scope : Scope
  c_bar : Constant  Value=3.45
  Aerodynamic Force : Outport
  Aerodynamic moment : Outport  Port=2
  wires:
  dynamic pressure/1 -> F_y/1, L/4, N/1, M/3, F_z/1, F_x/1
  Bus Element In/1 -> F_x/2
  S/1 -> F_x/3, L/1, N/2, M/4, F_z/3, F_y/3
  Bus Element In1/1 -> F_y/2
  Bus Element In2/1 -> F_z/2
  c_bar/1 -> M/2
  Bus Element In3/1 -> L/2
  Bus Element In4/1 -> M/1
  Bus Element In5/1 -> N/4
  B/1 -> N/3, L/3
  F_x/1 -> Force/1
  F_y/1 -> Force/2
  F_z/1 -> Force/3
  L/1 -> Moment/1  "L"
  M/1 -> Moment/2  "M"
  N/1 -> Moment/3  "N"
  Force/1 -> Aerodynamic Force/1
  Moment/1 -> Scope/1, Aerodynamic moment/1

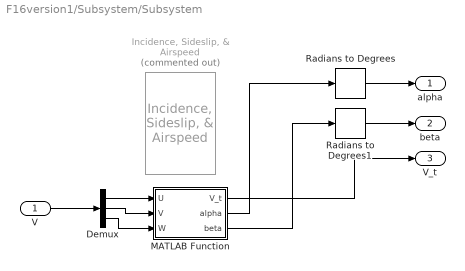
== system F16version1/Subsystem/Subsystem ==
  V : Inport
  Demux : Demux  Outputs=3
  "Incidence, Sideslip, & Airspeed" : aerolibasang/Incidence, Sideslip, & Airspeed  Commented=on
  MATLAB Function : MATLAB Function  TreatAsAtomicUnit=on
  Radians to Degrees : simulink_extras/Transformations/Radians to Degrees
  Radians to Degrees1 : simulink_extras/Transformations/Radians to Degrees
  alpha : Outport
  beta : Outport  Port=2
  V_t : Outport  Port=3
  wires:
  V/1 -> Demux/1
  Demux/1 -> MATLAB Function/1(U)
  Demux/2 -> MATLAB Function/2(V)
  Demux/3 -> MATLAB Function/3(W)
  Radians to Degrees/1 -> alpha/1
  Radians to Degrees1/1 -> beta/1
  MATLAB Function/3(beta) -> Radians to Degrees1/1
  MATLAB Function/2(alpha) -> Radians to Degrees/1
  MATLAB Function/1(V_t) -> V_t/1

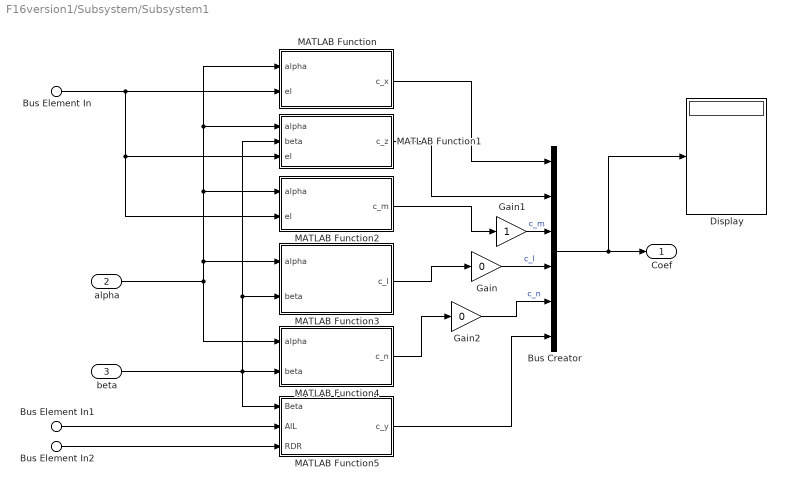
== system F16version1/Subsystem/Subsystem1 ==
  Bus Element In : Inport  PortName=ActuatorCmds  Element=Elevator
  Bus Element In1 : Inport  PortName=ActuatorCmds  Element=Aileron
  Bus Element In2 : Inport  PortName=ActuatorCmds  Element=Rudder
  alpha : Inport  Port=2
  beta : Inport  Port=3
  Bus Creator : BusCreator  Inputs=6
  Display : Display
  Gain : Gain  Gain=0
  Gain1 : Gain
  Gain2 : Gain  Gain=0
  MATLAB Function : MATLAB Function  TreatAsAtomicUnit=on
  MATLAB Function1 : MATLAB Function  TreatAsAtomicUnit=on
  MATLAB Function2 : MATLAB Function  TreatAsAtomicUnit=on
  MATLAB Function3 : MATLAB Function  TreatAsAtomicUnit=on
  MATLAB Function4 : MATLAB Function  TreatAsAtomicUnit=on
  MATLAB Function5 : MATLAB Function  TreatAsAtomicUnit=on
  Coef : Outport
  wires:
  Bus Element In1/1 -> MATLAB Function5/2(AIL)
  Bus Element In2/1 -> MATLAB Function5/3(RDR)
  Bus Element In/1 -> MATLAB Function/2(el), MATLAB Function1/3(el), MATLAB Function2/2(el)
  alpha/1 -> MATLAB Function3/1(alpha), MATLAB Function2/1(alpha), MATLAB Function/1(alpha), MATLAB Function1/1(alpha), MATLAB Function4/1(alpha)
  beta/1 -> MATLAB Function5/1(Beta), MATLAB Function1/2(beta), MATLAB Function3/2(beta), MATLAB Function4/2(beta)
  MATLAB Function/1(c_x) -> Bus Creator/1
  MATLAB Function1/1(c_z) -> Bus Creator/2
  MATLAB Function2/1(c_m) -> Gain1/1
  MATLAB Function4/1(c_n) -> Gain2/1
  MATLAB Function5/1(c_y) -> Bus Creator/6
  Bus Creator/1 -> Display/1, Coef/1
  MATLAB Function3/1(c_l) -> Gain/1
  Gain/1 -> Bus Creator/4  "c_l"
  Gain1/1 -> Bus Creator/3  "c_m"
  Gain2/1 -> Bus Creator/5  "c_n"

== matlab function F16version1/MATLAB Function2 ==
  data: alpha input; c_m output; el input
function c_m = compute_cm_fixed(alpha, el)
    % Embedded data
    data_CM_updated_data_full = [
        0.205, 0.168, 0.186, 0.196, 0.213, 0.251, 0.245, 0.238, 0.252, 0.231, 0.198, 0.192;
        0.081, 0.077, 0.107, 0.110, 0.110, 0.141, 0.127, 0.119, 0.133, 0.108, 0.081, 0.093;
        -0.046, -0.020, -0.009, -0.005, -0.006, 0.010, 0.006, -0.001, 0.014, 0.000, -0.013, 0.032;
        -0.174, -0.145, -0.121, -0.127, -0.129, -0.102, -0.097, -0.113, -0.087, -0.084, -0.069, -0.006;
        -0.259, -0.202, -0.184, -0.193, -0.199, -0.150, -0.160, -0.167, -0.104, -0.076, -0.041, -0.005
    ];

    % Map Alpha and EL into indices and interpolate
    scaled_alpha = 0.2 * alpha;
    k = floor(scaled_alpha);
    k = max(-2, min(k, 8)); % Constrain within bounds
    da = scaled_alpha - k;
    l = k + sign(1.1 * da);
    l = max(-1, min(l, 8)); % Constrain within bounds

    % Adjust indices for MATLAB (1-based indexing)
    k_index = k + 3;
    l_index = l + 3;

    scaled_el = el / 12.5;
    m = floor(scaled_el);
    m = max(-2, min(m, 2)); % Constrain within bounds
    de = scaled_el - m;
    n = m + sign(1.1 * de);
    n = max(-2, min(n, 2)); % Constrain within bounds

    % Adjust indices for MATLAB (1-based indexing)
    m_index = m + 3;
    n_index = n + 3;

    % Interpolate values
    t = data_CM_updated_data_full(m_index, k_index);
    u = data_CM_updated_data_full(n_index, k_index);
    v = t + abs(da) * (data_CM_updated_data_full(m_index, l_index) - t);
    w = u + abs(da) * (data_CM_updated_data_full(n_index, l_index) - u);

    % Final interpolation
    c_m = v + (w - v) * abs(de);
end

== matlab function F16version1/MATLAB Function3 ==
  data: alpha input; c_l output; beta input
function c_l = compute_cl_fixed(alpha, beta)
    % Embedded data
    data_CL_updated_data_full = [
        -0.001, -0.004, -0.008, -0.012, -0.016, -0.019, -0.020, -0.020, -0.015, -0.008, -0.013, -0.015;
        -0.003, -0.009, -0.017, -0.024, -0.030, -0.034, -0.040, -0.037, -0.016, -0.002, -0.010, -0.019;
        -0.001, -0.010, -0.020, -0.030, -0.039, -0.044, -0.050, -0.049, -0.023, -0.006, -0.014, -0.027;
        0.000, -0.010, -0.022, -0.034, -0.047, -0.046, -0.059, -0.061, -0.033, -0.036, -0.035, -0.035;
        0.007, -0.010, -0.023, -0.034, -0.049, -0.046, -0.068, -0.071, -0.060, -0.058, -0.062, -0.059;
        0.009, -0.011, -0.023, -0.037, -0.050, -0.047, -0.074, -0.079, -0.091, -0.076, -0.077, -0.076
    ];

    % Scale and map alpha into indices
    scaled_alpha = 0.2 * alpha;
    k = floor(scaled_alpha);                  % Find lower index
    k = max(-2, min(k, 8));                   % Constrain within bounds
    da = scaled_alpha - k;                    % Fractional part for interpolation
    l = k + sign(1.1 * da);                   % Find upper index
    l = max(-2, min(l, 8));                   % Constrain within bounds

    % Adjust indices for MATLAB (1-based indexing)
    k_index = k + 3;                          % Shift index for 1-based indexing
    l_index = l + 3;                          % Shift index for 1-based indexing

    % Scale and map beta into indices
    scaled_beta = 0.2 * abs(beta);
    m = floor(scaled_beta);                   % Find lower index
    m = max(0, min(m, 5));                    % Constrain within bounds
    db = scaled_beta - m;                     % Fractional part for interpolation
    n = m + sign(1.1 * db);                   % Find upper index
    n = max(0, min(n, 5));                    % Constrain within bounds

    % Adjust indices for MATLAB (1-based indexing)
    m_index = m + 1;                          % Shift index for 1-based indexing
    n_index = n + 1;                          % Shift index for 1-based indexing

    % Interpolation in the alpha dimension
    t = data_CL_updated_data_full(m_index, k_index); % Lower beta, lower alpha
    u = data_CL_updated_data_full(n_index, k_index); % Upper beta, lower alpha
    v = t + abs(da) * (data_CL_updated_data_full(m_index, l_index) - t); % Lower beta, interpolated alpha
    w = u + abs(da) * (data_CL_updated_data_full(n_index, l_index) - u); % Upper beta, interpolated alpha

    % Interpolation in the beta dimension
    c_l = v + (w - v) * abs(db);              % Final interpolated value
end

== matlab function F16version1/Subsystem/Subsystem1/MATLAB Function ==
  data: alpha input; c_x output; el input
function c_x = compute_cx_fixed(alpha, el)
    data = [
    -0.099, -0.081, -0.081, -0.063, -0.025, 0.044, 0.097, 0.113, 0.145, 0.167, 0.174, 0.166;
    -0.048, -0.038, -0.040, -0.021, 0.016, 0.083, 0.127, 0.137, 0.162, 0.177, 0.179, 0.167;
    -0.022, -0.020, -0.021, -0.004, 0.032, 0.094, 0.128, 0.130, 0.154, 0.161, 0.155, 0.138;
    -0.040, -0.038, -0.039, -0.025, 0.006, 0.062, 0.087, 0.085, 0.100, 0.110, 0.104, 0.091;
    -0.083, -0.073, -0.076, -0.072, -0.046, 0.012, 0.024, 0.025, 0.043, 0.053, 0.047, 0.040
    ];
    % Scale Alpha and EL
    scaled_alpha = 0.2 * alpha;
    k = floor(scaled_alpha);
    k = max(-2, min(k, 8)); % Constrain within bounds
    da = scaled_alpha - k;
    l = k + sign(1.1 * da);
    l = max(-2, min(l, 8)); % Constrain within bounds

    % Adjust indices for 1-based indexing
    k_index = k + 3; % MATLAB 1-based (add 3 instead of 2 for [-2, 8])
    l_index = l + 3;

    % Scale EL
    scaled_el = el / 12.5;
    m = floor(scaled_el);
    m = max(-2, min(m, 2)); % Constrain within bounds
    de = scaled_el - m;
    n = m + sign(1.1 * de);
    n = max(-2, min(n, 2)); % Constrain within bounds

    % Adjust indices for 1-based indexing
    m_index = m + 3; % MATLAB 1-based (add 3 instead of 2 for [-2, 2])
    n_index = n + 3;

    % Ensure indices are within valid ranges
    assert(m_index >= 1 && m_index <= size(data, 1), 'm_index out of bounds');
    assert(n_index >= 1 && n_index <= size(data, 1), 'n_index out of bounds');
    assert(k_index >= 1 && k_index <= size(data, 2), 'k_index out of bounds');
    assert(l_index >= 1 && l_index <= size(data, 2), 'l_index out of bounds');

    % Interpolate values
    t = data(m_index, k_index); % Top-left
    u = data(n_index, k_index); % Bottom-left
    v = t + abs(da) * (data(m_index, l_index) - t); % Interpolation along top row
    w = u + abs(da) * (data(n_index, l_index) - u); % Interpolation along bottom row
    c_x = v + (w - v) * abs(de); % Final interpolation
end

== matlab function F16version1/MATLAB Function4 ==
  data: alpha input; c_n output; beta input
function c_n = compute_cn_fixed(alpha, beta)
    % Embedded data
    data_CN_updated_data_full = [
        0.018, 0.019, 0.018, 0.019, 0.019, 0.018, 0.013, 0.007, 0.004, -0.014, -0.017, -0.033;
        0.038, 0.042, 0.042, 0.042, 0.043, 0.039, 0.030, 0.017, 0.004, -0.035, -0.047, -0.057;
        0.056, 0.057, 0.059, 0.058, 0.058, 0.053, 0.032, 0.012, 0.002, -0.046, -0.071, -0.073;
        0.064, 0.077, 0.076, 0.074, 0.073, 0.057, 0.029, 0.007, 0.012, -0.034, -0.065, -0.041;
        0.074, 0.086, 0.093, 0.089, 0.080, 0.062, 0.049, 0.022, 0.028, -0.012, -0.002, -0.013;
        0.079, 0.090, 0.106, 0.106, 0.096, 0.080, 0.068, 0.030, 0.064, 0.015, 0.011, -0.001
    ];

    % Scale and map alpha into indices
    scaled_alpha = 0.2 * alpha;
    k = floor(scaled_alpha);                  % Find lower index
    k = max(-2, min(k, 8));                   % Constrain within bounds
    da = scaled_alpha - k;                    % Fractional part for interpolation
    l = k + sign(1.1 * da);                   % Find upper index
    l = max(-2, min(l, 8));                   % Constrain within bounds

    % Adjust indices for MATLAB (1-based indexing)
    k_index = k + 3;                          % Shift index for 1-based indexing
    l_index = l + 3;                          % Shift index for 1-based indexing

    % Scale and map beta into indices
    scaled_beta = 0.2 * abs(beta);
    m = floor(scaled_beta);                   % Find lower index
    m = max(0, min(m, 5));                    % Constrain within bounds
    db = scaled_beta - m;                     % Fractional part for interpolation
    n = m + sign(1.1 * db);                   % Find upper index
    n = max(0, min(n, 5));                    % Constrain within bounds

    % Adjust indices for MATLAB (1-based indexing)
    m_index = m + 1;                          % Shift index for 1-based indexing
    n_index = n + 1;                          % Shift index for 1-based indexing

    % Interpolation in the alpha dimension
    t = data_CN_updated_data_full(m_index, k_index); % Lower beta, lower alpha
    u = data_CN_updated_data_full(n_index, k_index); % Upper beta, lower alpha
    v = t + abs(da) * (data_CN_updated_data_full(m_index, l_index) - t); % Lower beta, interpolated alpha
    w = u + abs(da) * (data_CN_updated_data_full(n_index, l_index) - u); % Upper beta, interpolated alpha

    % Interpolation in the beta dimension
    c_n = v + (w - v) * abs(db);              % Final interpolated value
end

== matlab function F16version1/MATLAB Function5 ==
  data: Beta input; c_y output; AIL input; RDR input
function c_y = compute_C_Y(Beta, AIL, RDR)
    % Compute C_Y based on Beta, AIL, and RDR
    c_y = (-0.02) * Beta + (0.021) * (AIL / 20.0) + (0.086) * (RDR / 30.0);
end

== matlab function F16version1/Subsystem/Subsystem1/MATLAB Function1 ==
  data: alpha input; c_z output; beta input; el input


function c_z = compute_cz(alpha, beta, el)
    data_CZ_updated_data_full = [
    0.770, 0.241, -0.100, -0.416, -0.731, -1.053, ...
    -1.366, -1.646, -1.917, -2.120, -2.248, -2.229
    ];
    
    % Map Alpha into indices and interpolate
    scaled_alpha = 0.2 * alpha;
    k = floor(scaled_alpha);
    k = max(-2, min(k, 8)); % Constrain within bounds
    da = scaled_alpha - k;
    l = k + sign(1.1 * da);
    l = max(-1, min(l, 8)); % Constrain within bounds

    % Adjust index for MATLAB (1-based indexing)
    k_index = k + 3;
    l_index = l + 3;

    % Calculate 's' using the provided formula
    s = data_CZ_updated_data_full(k_index) + abs(da) * ...
        (data_CZ_updated_data_full(l_index) - data_CZ_updated_data_full(k_index));
    c_z = s * (1 - (beta / 57.3)^2) - 0.19 * (el / 25.0);
end
